simulink model "DR_Backlog_Model"  (R2026a)
settings: Solver=VariableStepAuto  StopTime=28800
Description:
  | CAMP-DAY BACKLOG SIMULATOR (Track B). Question: at what arrival rate does the doctor queue start growing? Flow (left to right): hourly arrivals -> per-second -> AI delay (2.5s) -> compare against doctor service (1/105 patients per sec = 5 min per referable x 35 percent referable) -> integrate the difference, floored at zero. Toy: averaged flow, single doctor, flat arrivals. See simulink/README_TRACKB.md.
settings Model: Creator=SHIVANYA SALES  LastModifiedBy=SHIVANYA SALES

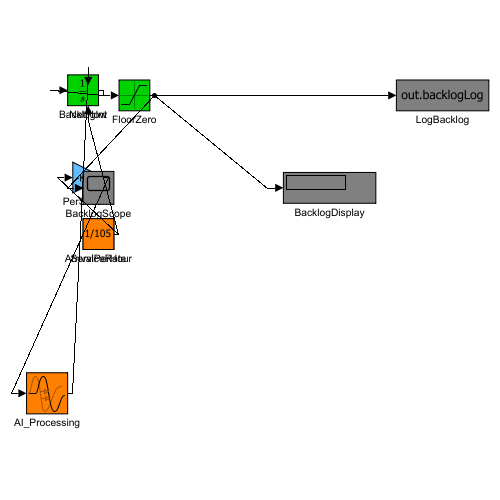
[thumbnail: Simulink's stored preview of the top-level diagram]
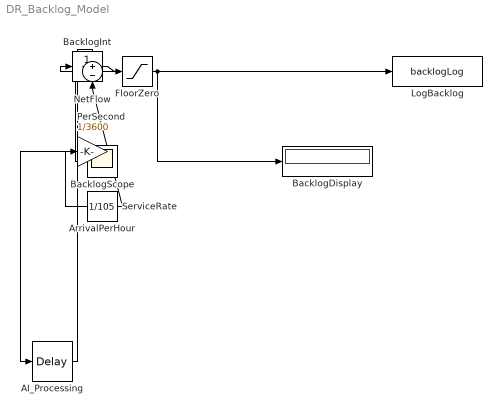
== system DR_Backlog_Model ==
  AI_Processing : TransportDelay  DelayTime=2.5
  ArrivalPerHour : Constant  Description=Patients arriving per hour. Edit me: 20 = normal day, 40 = stress day.  Value=20
  BacklogDisplay : Display
  BacklogInt : Integrator  Description=Running total of (arrivals minus served). This is THE backlog.
  BacklogScope : Scope
      settings: Description=THE RESULT: flat zero = camp copes; rising ramp = camp breaks.
  FloorZero : Saturate  Description=A queue cannot go negative: clips at zero.  UpperLimit=inf  LowerLimit=0
  LogBacklog : ToWorkspace  VariableName=backlogLog  SampleTime=-1
  NetFlow : Sum  Inputs=+-
  PerSecond : Gain  Gain=1/3600
  ServiceRate : Constant  Description=Doctor speed: 1 patient per 105 sec average (5 min per referable x 35 percent referable = 34.3 patients per hour).  Value=1/105
  wires:
  ArrivalPerHour/1 -> PerSecond/1
  PerSecond/1 -> AI_Processing/1
  AI_Processing/1 -> NetFlow/1
  ServiceRate/1 -> NetFlow/2
  NetFlow/1 -> BacklogInt/1
  BacklogInt/1 -> FloorZero/1
  FloorZero/1 -> BacklogScope/1, BacklogDisplay/1, LogBacklog/1
